simulink model "untitled6"  (R2018b)
settings: Solver=VariableStepAuto  StartTime=0.0  StopTime=inf  RelTol=1e-3
libraries: commdigbbndpm3 x2, commchan3 x1, commrandsrc3 x1, commsink2 x1
settings Model: Creator=nhat  LastModifiedBy=nhat

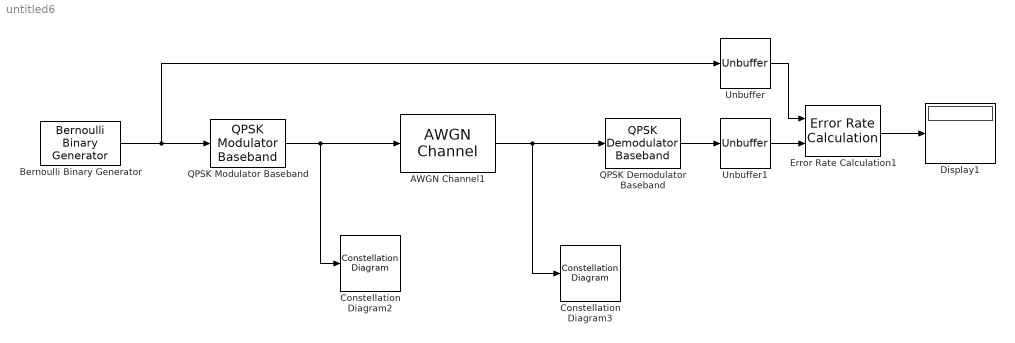
== system untitled6 ==
  AWGN Channel1 : commchan3/AWGN Channel  InputProcessing=Columns as channels (frame based)  seed=67  noiseMode="Signal to noise ratio  (Eb/No)"  EbNodB=10  EsNodB=5  SNRdB=10  bitsPerSym=2  Ps=1  Tsym=1/1000  variance=1
  Bernoulli Binary Generator : commrandsrc3/Bernoulli Binary Generator  ProbabilityOfZero=0.5  SeedSource=Auto  Seed=0  SampleTime=1/2000  SamplesPerFrame=100  OutputDataType=double  SimulateUsing=Interpreted execution
  Constellation Diagram2 : ConstellationDiagram
  Constellation Diagram3 : ConstellationDiagram
  Display1 : Display
  Error Rate Calculation1 : commsink2/Error Rate Calculation  N=0  st_delay=0  cp_mode=Entire frame  subframe=[]  PMode=Port  WsName=ErrorVec  RsMode2=off  stop=on  numErr=100  maxBits=1e6
  QPSK Demodulator Baseband : commdigbbndpm3/QPSK Demodulator Baseband  OutType=Bit  DecType=Hard decision  VarSource=Dialog  Variance=1  Dec=Gray  Ph=pi/4  outDtype1=Inherit via internal rule  outDtype2=Inherit via internal rule  derotateFactorWordLen=16  derotateFactorDataTypeStr=Inherit: Same word length as input  derotateFactorLastDataTypeStr=Inherit: Same word length as input
  QPSK Modulator Baseband : commdigbbndpm3/QPSK Modulator Baseband  InType=Bit  Enc=Gray  Ph=pi/4  outDtype=double  outWordLen=16  outUDDataType=sfix(16)  outFracLenMode=Best precision  outFracLen=15  outDataTypeStr=double  outLastDataTypeStr=double
  Unbuffer : Unbuffer
  Unbuffer1 : Unbuffer
  wires:
  Unbuffer/1 -> Error Rate Calculation1/1
  QPSK Modulator Baseband/1 -> Constellation Diagram2/1, AWGN Channel1/1
  Error Rate Calculation1/1 -> Display1/1
  Bernoulli Binary Generator/1 -> Unbuffer/1, QPSK Modulator Baseband/1
  AWGN Channel1/1 -> QPSK Demodulator Baseband/1, Constellation Diagram3/1
  QPSK Demodulator Baseband/1 -> Unbuffer1/1
  Unbuffer1/1 -> Error Rate Calculation1/2
